simulink model "Application_Problem_Solution"  (R2018b)
settings: Solver=VariableStepAuto  StartTime=0.0  StopTime=6300  FixedStep=0.1  RelTol=1e-3  EnableMultiTasking=on
StopFcn:
  | if sum(Diagnostic_Decision_PV_1)>0
  | f = msgbox('Failure in PV 1');
  | end
  | 
  | if sum(Diagnostic_Decision_PV_2)>0
  | f = msgbox('Failure in PV 2');
  | end
  | 
  | if sum(Diagnostic_Decision_PV_3)>0
  | f = msgbox('Failure in PV 3');
  | end
  | 
  | if sum(Diagnostic_Decision_PV_4)>0
  | f = msgbox('Failure in PV 4');
  | end
  | 
  | if sum(Diagnostic_Decision_PV_5)>0
  | f = msgbox('Failure in PV 5');
  | end
  | 
  | if sum(Diagnostic_Decision_PV_6)>0
  | f = msgbox('Failure in PV 6');
  | end
  | 
  | if sum(Diagnostic_Decision_PV_7)>0
  | f = msgbox('Failure in PV 7');
  | end
  | 
  | if sum(Diagnostic_Decision_PV_8)>0
  | f = msgbox('Failure in PV 8');
  | end
  | 
  | if sum(Diagnostic_Decision_PV_9)>0
  | f = msgbox('Failure in PV 9');
  | end
  | 
  | if sum(Diagnostic_Decision_PV_10)>0
  | f = msgbox('Failure in PV 10');
  | end
values from neighbouring files (symbols this model uses):
  C1_LUT = [1913.6 4625.7 23306 10736 18036 12251 9022.9 12447 18872 40764 18721 33630 ... (21 elements, 7x3)]    [model_data_application.mat]
  Capacity_LUT = [28.0081 27.625 27.6392]    [model_data_application.mat]
  cell_Cp_heat = 810.5328    [model_data_application.mat]
  cell_mass = 1    [model_data_application.mat]
  Em_LUT = [3.4966 3.5519 3.6183 3.7066 3.9131 4.0748 4.1923 3.5057 3.566 3.6337 3.7127 3.9259 ... (21 elements, 7x3)]    [model_data_application.mat]
  Qe_init = 3.6845    [model_data_application.mat]
  R0_LUT = [0.0117 0.011 0.0114 0.0107 0.0107 0.0113 0.0116 0.0085 0.0085 0.0087 0.0082 0.0083 ... (21 elements, 7x3)]    [model_data_application.mat]
  R1_LUT = [0.0109 0.0069 0.0047 0.0034 0.0033 0.0033 0.0028 0.0029 0.0024 0.0026 0.0016 0.0023 ... (21 elements, 7x3)]    [model_data_application.mat]
  SOC_LUT = [0 0.1 0.25 0.5 0.75 0.9 1]    [model_data_application.mat]
  T_init = 293.15    [model_data_application.mat]
  Temperature_LUT = [278.15 293.15 313.15]    [model_data_application.mat]
undefined symbols (not defined in the file or in its folder): DiscIntNeverNeededParam
libraries: elec_lib x450, fl_lib x121, LiBatteryElements_lib x40, nesl_utility x32, simulink x10
(part 1 of 3)
settings Model: Creator=Sanjay Lodwal  LastModifiedBy=user
settings DataIOCC: LimitDataPoints=on  SaveFormat=Array
settings OptimizationCC: LifeSpan=inf
settings DebuggingCC: UnderspecifiedInitializationDetection=Classic  MergeDetectMultiDrivingBlocksExec=none  SolverPrmCheckMsg=warning  StateNameClashWarn=warning  SFUnexpectedBacktrackingDiag=warning  SFNoUnconditionalDefaultTransitionDiag=warning  SFExecutionAtInitializationDiag=none
settings HardwareCC: ProdBitPerPointer=32  ProdBitPerSizeT=32  ProdBitPerPtrDiffT=32  ProdLargestAtomicFloat=None  ProdIntDivRoundTo=Undefined  ProdEndianess=Unspecified  ProdWordSize=32  ProdHWDeviceType=32-bit Generic
settings ModelReferenceCC: PropagateSignalLabelsOutOfModel=off
settings SFSimCC: SimUseLocalCustomCode=off
settings RTWCC: RTWUseLocalCustomCode=off
settings CodeAppCC: StateflowObjectComments=on
settings GRTTargetCC: TargetLangStandard=C89/C90 (ANSI)  GeneratePreprocessorConditionals=Disable all
settings ConfigComp: CovMetricSettings=dw  CovHtmlReporting=on  CovSaveCumulativeToWorkspaceVar=on  CovSaveSingleToWorkspaceVar=on  CovExternalEMLEnable=off
settings SimscapeCC: SimscapeNormalizeSystem=off

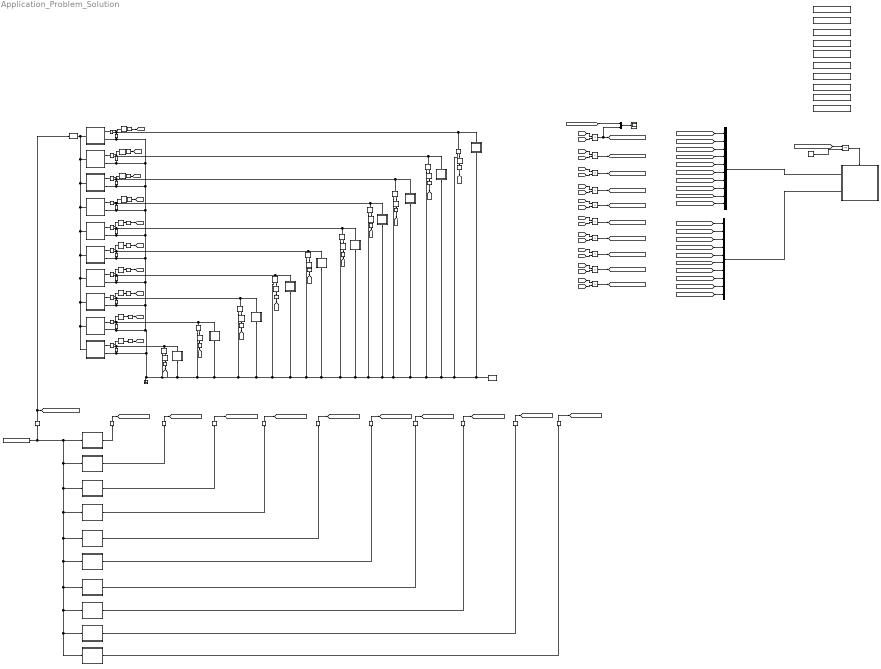
== system Application_Problem_Solution ==
  Battery1 : Subsystem  mask(Lithium cell (one RC-branch equivalent circuit)){Qe_init=Qe_init, T_init=T_init, Capacity_LUT=Capacity_LUT, Em_LUT=Em_LUT, R0_LUT=R0_LUT, R1_LUT=R1_LUT, C1_LUT=C1_LUT, cell_mass=cell_mass, cell_Cp_heat=cell_Cp_heat, SOC_LUT=SOC_LUT, Temperature_LUT=Temperature_LUT}
      mask prompts: Qe_init "Initial charge deficit (A*hr)"; T_init "Initial cell temperature (K)"; Capacity_LUT "Capacity (A*hr, 1xN table)"; Em_LUT "Em open-circuit voltage (volts, MxN table)"; R0_LUT "R0 terminal resistance (ohms, MxN table)"; R1_LUT "R1 resistance (ohms, MxN table)"; C1_LUT "C1 capacitance (farads, MxN table)"; cell_mass "Cell mass (kg)"; cell_Cp_heat "Cell specific heat (J/kg/K)"; SOC_LUT "SOC table breakpoints (Mx1 array)"; Temperature_LUT "Temperature table breakpoints (K, 1xN array)"
      mask DialogControl ParameterTabVar0 Prompt: Initial Conditions
      mask DialogControl ParameterTabVar01 Prompt: Electrical
      mask DialogControl ParameterTabVar012 Prompt: Thermal
      mask DialogControl ParameterTabVar0123 Prompt: Table Breakpoints
      mask Display: image('battery.jpg')
  Battery10 : Subsystem  mask(Lithium cell (one RC-branch equivalent circuit)){Qe_init=Qe_init, T_init=T_init, Capacity_LUT=Capacity_LUT, Em_LUT=Em_LUT, R0_LUT=R0_LUT, R1_LUT=R1_LUT, C1_LUT=C1_LUT, cell_mass=cell_mass, cell_Cp_heat=cell_Cp_heat, SOC_LUT=SOC_LUT, Temperature_LUT=Temperature_LUT}
      mask prompts: Qe_init "Initial charge deficit (A*hr)"; T_init "Initial cell temperature (K)"; Capacity_LUT "Capacity (A*hr, 1xN table)"; Em_LUT "Em open-circuit voltage (volts, MxN table)"; R0_LUT "R0 terminal resistance (ohms, MxN table)"; R1_LUT "R1 resistance (ohms, MxN table)"; C1_LUT "C1 capacitance (farads, MxN table)"; cell_mass "Cell mass (kg)"; cell_Cp_heat "Cell specific heat (J/kg/K)"; SOC_LUT "SOC table breakpoints (Mx1 array)"; Temperature_LUT "Temperature table breakpoints (K, 1xN array)"
      mask DialogControl ParameterTabVar0 Prompt: Initial Conditions
      mask DialogControl ParameterTabVar01 Prompt: Electrical
      mask DialogControl ParameterTabVar012 Prompt: Thermal
      mask DialogControl ParameterTabVar0123 Prompt: Table Breakpoints
      mask Display: image('battery.jpg')
  Battery2 : Subsystem  mask(Lithium cell (one RC-branch equivalent circuit)){Qe_init=Qe_init, T_init=T_init, Capacity_LUT=Capacity_LUT, Em_LUT=Em_LUT, R0_LUT=R0_LUT, R1_LUT=R1_LUT, C1_LUT=C1_LUT, cell_mass=cell_mass, cell_Cp_heat=cell_Cp_heat, SOC_LUT=SOC_LUT, Temperature_LUT=Temperature_LUT}
      mask prompts: Qe_init "Initial charge deficit (A*hr)"; T_init "Initial cell temperature (K)"; Capacity_LUT "Capacity (A*hr, 1xN table)"; Em_LUT "Em open-circuit voltage (volts, MxN table)"; R0_LUT "R0 terminal resistance (ohms, MxN table)"; R1_LUT "R1 resistance (ohms, MxN table)"; C1_LUT "C1 capacitance (farads, MxN table)"; cell_mass "Cell mass (kg)"; cell_Cp_heat "Cell specific heat (J/kg/K)"; SOC_LUT "SOC table breakpoints (Mx1 array)"; Temperature_LUT "Temperature table breakpoints (K, 1xN array)"
      mask DialogControl ParameterTabVar0 Prompt: Initial Conditions
      mask DialogControl ParameterTabVar01 Prompt: Electrical
      mask DialogControl ParameterTabVar012 Prompt: Thermal
      mask DialogControl ParameterTabVar0123 Prompt: Table Breakpoints
      mask Display: image('battery.jpg')
  Battery3 : Subsystem  mask(Lithium cell (one RC-branch equivalent circuit)){Qe_init=Qe_init, T_init=T_init, Capacity_LUT=Capacity_LUT, Em_LUT=Em_LUT, R0_LUT=R0_LUT, R1_LUT=R1_LUT, C1_LUT=C1_LUT, cell_mass=cell_mass, cell_Cp_heat=cell_Cp_heat, SOC_LUT=SOC_LUT, Temperature_LUT=Temperature_LUT}
      mask prompts: Qe_init "Initial charge deficit (A*hr)"; T_init "Initial cell temperature (K)"; Capacity_LUT "Capacity (A*hr, 1xN table)"; Em_LUT "Em open-circuit voltage (volts, MxN table)"; R0_LUT "R0 terminal resistance (ohms, MxN table)"; R1_LUT "R1 resistance (ohms, MxN table)"; C1_LUT "C1 capacitance (farads, MxN table)"; cell_mass "Cell mass (kg)"; cell_Cp_heat "Cell specific heat (J/kg/K)"; SOC_LUT "SOC table breakpoints (Mx1 array)"; Temperature_LUT "Temperature table breakpoints (K, 1xN array)"
      mask DialogControl ParameterTabVar0 Prompt: Initial Conditions
      mask DialogControl ParameterTabVar01 Prompt: Electrical
      mask DialogControl ParameterTabVar012 Prompt: Thermal
      mask DialogControl ParameterTabVar0123 Prompt: Table Breakpoints
      mask Display: image('battery.jpg')
  Battery4 : Subsystem  mask(Lithium cell (one RC-branch equivalent circuit)){Qe_init=Qe_init, T_init=T_init, Capacity_LUT=Capacity_LUT, Em_LUT=Em_LUT, R0_LUT=R0_LUT, R1_LUT=R1_LUT, C1_LUT=C1_LUT, cell_mass=cell_mass, cell_Cp_heat=cell_Cp_heat, SOC_LUT=SOC_LUT, Temperature_LUT=Temperature_LUT}
      mask prompts: Qe_init "Initial charge deficit (A*hr)"; T_init "Initial cell temperature (K)"; Capacity_LUT "Capacity (A*hr, 1xN table)"; Em_LUT "Em open-circuit voltage (volts, MxN table)"; R0_LUT "R0 terminal resistance (ohms, MxN table)"; R1_LUT "R1 resistance (ohms, MxN table)"; C1_LUT "C1 capacitance (farads, MxN table)"; cell_mass "Cell mass (kg)"; cell_Cp_heat "Cell specific heat (J/kg/K)"; SOC_LUT "SOC table breakpoints (Mx1 array)"; Temperature_LUT "Temperature table breakpoints (K, 1xN array)"
      mask DialogControl ParameterTabVar0 Prompt: Initial Conditions
      mask DialogControl ParameterTabVar01 Prompt: Electrical
      mask DialogControl ParameterTabVar012 Prompt: Thermal
      mask DialogControl ParameterTabVar0123 Prompt: Table Breakpoints
      mask Display: image('battery.jpg')
  Battery5 : Subsystem  mask(Lithium cell (one RC-branch equivalent circuit)){Qe_init=Qe_init, T_init=T_init, Capacity_LUT=Capacity_LUT, Em_LUT=Em_LUT, R0_LUT=R0_LUT, R1_LUT=R1_LUT, C1_LUT=C1_LUT, cell_mass=cell_mass, cell_Cp_heat=cell_Cp_heat, SOC_LUT=SOC_LUT, Temperature_LUT=Temperature_LUT}
      mask prompts: Qe_init "Initial charge deficit (A*hr)"; T_init "Initial cell temperature (K)"; Capacity_LUT "Capacity (A*hr, 1xN table)"; Em_LUT "Em open-circuit voltage (volts, MxN table)"; R0_LUT "R0 terminal resistance (ohms, MxN table)"; R1_LUT "R1 resistance (ohms, MxN table)"; C1_LUT "C1 capacitance (farads, MxN table)"; cell_mass "Cell mass (kg)"; cell_Cp_heat "Cell specific heat (J/kg/K)"; SOC_LUT "SOC table breakpoints (Mx1 array)"; Temperature_LUT "Temperature table breakpoints (K, 1xN array)"
      mask DialogControl ParameterTabVar0 Prompt: Initial Conditions
      mask DialogControl ParameterTabVar01 Prompt: Electrical
      mask DialogControl ParameterTabVar012 Prompt: Thermal
      mask DialogControl ParameterTabVar0123 Prompt: Table Breakpoints
      mask Display: image('battery.jpg')
  Battery6 : Subsystem  mask(Lithium cell (one RC-branch equivalent circuit)){Qe_init=Qe_init, T_init=T_init, Capacity_LUT=Capacity_LUT, Em_LUT=Em_LUT, R0_LUT=R0_LUT, R1_LUT=R1_LUT, C1_LUT=C1_LUT, cell_mass=cell_mass, cell_Cp_heat=cell_Cp_heat, SOC_LUT=SOC_LUT, Temperature_LUT=Temperature_LUT}
      mask prompts: Qe_init "Initial charge deficit (A*hr)"; T_init "Initial cell temperature (K)"; Capacity_LUT "Capacity (A*hr, 1xN table)"; Em_LUT "Em open-circuit voltage (volts, MxN table)"; R0_LUT "R0 terminal resistance (ohms, MxN table)"; R1_LUT "R1 resistance (ohms, MxN table)"; C1_LUT "C1 capacitance (farads, MxN table)"; cell_mass "Cell mass (kg)"; cell_Cp_heat "Cell specific heat (J/kg/K)"; SOC_LUT "SOC table breakpoints (Mx1 array)"; Temperature_LUT "Temperature table breakpoints (K, 1xN array)"
      mask DialogControl ParameterTabVar0 Prompt: Initial Conditions
      mask DialogControl ParameterTabVar01 Prompt: Electrical
      mask DialogControl ParameterTabVar012 Prompt: Thermal
      mask DialogControl ParameterTabVar0123 Prompt: Table Breakpoints
      mask Display: image('battery.jpg')
  Battery7 : Subsystem  mask(Lithium cell (one RC-branch equivalent circuit)){Qe_init=Qe_init, T_init=T_init, Capacity_LUT=Capacity_LUT, Em_LUT=Em_LUT, R0_LUT=R0_LUT, R1_LUT=R1_LUT, C1_LUT=C1_LUT, cell_mass=cell_mass, cell_Cp_heat=cell_Cp_heat, SOC_LUT=SOC_LUT, Temperature_LUT=Temperature_LUT}
      mask prompts: Qe_init "Initial charge deficit (A*hr)"; T_init "Initial cell temperature (K)"; Capacity_LUT "Capacity (A*hr, 1xN table)"; Em_LUT "Em open-circuit voltage (volts, MxN table)"; R0_LUT "R0 terminal resistance (ohms, MxN table)"; R1_LUT "R1 resistance (ohms, MxN table)"; C1_LUT "C1 capacitance (farads, MxN table)"; cell_mass "Cell mass (kg)"; cell_Cp_heat "Cell specific heat (J/kg/K)"; SOC_LUT "SOC table breakpoints (Mx1 array)"; Temperature_LUT "Temperature table breakpoints (K, 1xN array)"
      mask DialogControl ParameterTabVar0 Prompt: Initial Conditions
      mask DialogControl ParameterTabVar01 Prompt: Electrical
      mask DialogControl ParameterTabVar012 Prompt: Thermal
      mask DialogControl ParameterTabVar0123 Prompt: Table Breakpoints
      mask Display: image('battery.jpg')
  Battery8 : Subsystem  mask(Lithium cell (one RC-branch equivalent circuit)){Qe_init=Qe_init, T_init=T_init, Capacity_LUT=Capacity_LUT, Em_LUT=Em_LUT, R0_LUT=R0_LUT, R1_LUT=R1_LUT, C1_LUT=C1_LUT, cell_mass=cell_mass, cell_Cp_heat=cell_Cp_heat, SOC_LUT=SOC_LUT, Temperature_LUT=Temperature_LUT}
      mask prompts: Qe_init "Initial charge deficit (A*hr)"; T_init "Initial cell temperature (K)"; Capacity_LUT "Capacity (A*hr, 1xN table)"; Em_LUT "Em open-circuit voltage (volts, MxN table)"; R0_LUT "R0 terminal resistance (ohms, MxN table)"; R1_LUT "R1 resistance (ohms, MxN table)"; C1_LUT "C1 capacitance (farads, MxN table)"; cell_mass "Cell mass (kg)"; cell_Cp_heat "Cell specific heat (J/kg/K)"; SOC_LUT "SOC table breakpoints (Mx1 array)"; Temperature_LUT "Temperature table breakpoints (K, 1xN array)"
      mask DialogControl ParameterTabVar0 Prompt: Initial Conditions
      mask DialogControl ParameterTabVar01 Prompt: Electrical
      mask DialogControl ParameterTabVar012 Prompt: Thermal
      mask DialogControl ParameterTabVar0123 Prompt: Table Breakpoints
      mask Display: image('battery.jpg')
  Battery9 : Subsystem  mask(Lithium cell (one RC-branch equivalent circuit)){Qe_init=Qe_init, T_init=T_init, Capacity_LUT=Capacity_LUT, Em_LUT=Em_LUT, R0_LUT=R0_LUT, R1_LUT=R1_LUT, C1_LUT=C1_LUT, cell_mass=cell_mass, cell_Cp_heat=cell_Cp_heat, SOC_LUT=SOC_LUT, Temperature_LUT=Temperature_LUT}
      mask prompts: Qe_init "Initial charge deficit (A*hr)"; T_init "Initial cell temperature (K)"; Capacity_LUT "Capacity (A*hr, 1xN table)"; Em_LUT "Em open-circuit voltage (volts, MxN table)"; R0_LUT "R0 terminal resistance (ohms, MxN table)"; R1_LUT "R1 resistance (ohms, MxN table)"; C1_LUT "C1 capacitance (farads, MxN table)"; cell_mass "Cell mass (kg)"; cell_Cp_heat "Cell specific heat (J/kg/K)"; SOC_LUT "SOC table breakpoints (Mx1 array)"; Temperature_LUT "Temperature table breakpoints (K, 1xN array)"
      mask DialogControl ParameterTabVar0 Prompt: Initial Conditions
      mask DialogControl ParameterTabVar01 Prompt: Electrical
      mask DialogControl ParameterTabVar012 Prompt: Thermal
      mask DialogControl ParameterTabVar0123 Prompt: Table Breakpoints
      mask Display: image('battery.jpg')
  Current Sensor{,1..9} (10 alike) : fl_lib/Electrical/Electrical Sensors/Current Sensor
  Data Store Memory : DataStoreMemory  DataStoreName=Diagnostic_Decision_PV_1  ReadBeforeWriteMsg=warning  WriteAfterWriteMsg=warning  WriteAfterReadMsg=warning  ShowAdditionalParam=off
  Data Store Memory1 : DataStoreMemory  DataStoreName=Diagnostic_Decision_PV_2  ReadBeforeWriteMsg=warning  WriteAfterWriteMsg=warning  WriteAfterReadMsg=warning  ShowAdditionalParam=off
  Data Store Memory2 : DataStoreMemory  DataStoreName=Diagnostic_Decision_PV_3  ReadBeforeWriteMsg=warning  WriteAfterWriteMsg=warning  WriteAfterReadMsg=warning  ShowAdditionalParam=off
  Data Store Memory3 : DataStoreMemory  DataStoreName=Diagnostic_Decision_PV_4  ReadBeforeWriteMsg=warning  WriteAfterWriteMsg=warning  WriteAfterReadMsg=warning  ShowAdditionalParam=off
  Data Store Memory4 : DataStoreMemory  DataStoreName=Diagnostic_Decision_PV_5  ReadBeforeWriteMsg=warning  WriteAfterWriteMsg=warning  WriteAfterReadMsg=warning  ShowAdditionalParam=off
  Data Store Memory5 : DataStoreMemory  DataStoreName=Diagnostic_Decision_PV_6  ReadBeforeWriteMsg=warning  WriteAfterWriteMsg=warning  WriteAfterReadMsg=warning  ShowAdditionalParam=off
  Data Store Memory6 : DataStoreMemory  DataStoreName=Diagnostic_Decision_PV_7  ReadBeforeWriteMsg=warning  WriteAfterWriteMsg=warning  WriteAfterReadMsg=warning  ShowAdditionalParam=off
  Data Store Memory7 : DataStoreMemory  DataStoreName=Diagnostic_Decision_PV_8  ReadBeforeWriteMsg=warning  WriteAfterWriteMsg=warning  WriteAfterReadMsg=warning  ShowAdditionalParam=off
  Data Store Memory8 : DataStoreMemory  DataStoreName=Diagnostic_Decision_PV_9  ReadBeforeWriteMsg=warning  WriteAfterWriteMsg=warning  WriteAfterReadMsg=warning  ShowAdditionalParam=off
  Data Store Memory9 : DataStoreMemory  DataStoreName=Diagnostic_Decision_PV_10  ReadBeforeWriteMsg=warning  WriteAfterWriteMsg=warning  WriteAfterReadMsg=warning  ShowAdditionalParam=off
  Diagnostic Block : Subsystem  TreatAsAtomicUnit=on
  Diode{,1..9} (10 alike) : fl_lib/Electrical/Electrical Elements/Diode  Vf=0.6 V  Ron=0.3 Ohm  Goff=1e-8 1/Ohm  i_specify=off  i_priority=High  i=0 A  i_nominal_specify=off  i_nominal_unit=A  i_nominal_value=1  v_specify=off  v_priority=High  v=0 V  v_nominal_specify=off  v_nominal_unit=V  v_nominal_value=1
  Electrical Reference : fl_lib/Electrical/Electrical Elements/Electrical Reference
  Ir : FromWorkspace  VariableName=irradiance_measurement_8hrs  SampleTime=0
  Minimum Light Conditions : Constant  Value=500
  Mux : Mux  Inputs=2
  Mux1 : Mux  Inputs=10
  Mux2 : Mux  Inputs=10
  PS-Simulink Converter{1..20} (20 alike) : nesl_utility/PS-Simulink Converter  PhysicalDomain=network_engine_domain  SubClassName=ps_output  LeftPortType=input  RightPortType=output  PseudoPeriodic=off  Frequencies=[]  Unit=1  AffineConversion=off
  PV 1 Physical : Subsystem
      mask Display: image('PV_physical.png');
  PV 10 Physical : Subsystem
      mask Display: image('PV_physical.png');
  "PV 2 Physical " : Subsystem
      mask Display: image('PV_physical.png');
  PV 3 Physical : Subsystem
      mask Display: image('PV_physical.png');
  PV 4 Physical : Subsystem
      mask Display: image('PV_physical.png');
  PV 5 Physical : Subsystem
      mask Display: image('PV_physical.png');
  PV 6 Physical : Subsystem
      mask Display: image('PV_physical.png');
  PV 7 Physical : Subsystem
      mask Display: image('PV_physical.png');
  PV 8 Physical : Subsystem
      mask Display: image('PV_physical.png');
  PV 9 Physical : Subsystem
      mask Display: image('PV_physical.png');
  PV1 Digital Twin : Subsystem  mask{Isc=5.49, Voc=21.5, n=1.5, Rs=0, Ir0=1000, T=30}
      mask prompts: Isc "Short circuit current"; Voc "Open circuit voltage"; n "Quality factor, N"; Rs "Series resistance"; Ir0 "Reference irradiation"; T "Temperature"
      mask Display: image('PV1.jpg')
  PV10 Digital Twin : Subsystem  mask{Isc=5.49, Voc=21.5, n=1.5, Rs=0, Ir0=1000, T=30}
      mask prompts: Isc "Short circuit current"; Voc "Open circuit voltage"; n "Quality factor, N"; Rs "Series resistance"; Ir0 "Reference irradiation"; T "Temperature"
      mask Display: image('PV1.jpg')
  PV2 Digital Twin : Subsystem  mask{Isc=5.49, Voc=21.5, n=1.5, Rs=0, Ir0=1000, T=30}
      mask prompts: Isc "Short circuit current"; Voc "Open circuit voltage"; n "Quality factor, N"; Rs "Series resistance"; Ir0 "Reference irradiation"; T "Temperature"
      mask Display: image('PV1.jpg')
  "PV3 Digital Twin " : Subsystem  mask{Isc=5.49, Voc=21.5, n=1.5, Rs=0, Ir0=1000, T=30}
      mask prompts: Isc "Short circuit current"; Voc "Open circuit voltage"; n "Quality factor, N"; Rs "Series resistance"; Ir0 "Reference irradiation"; T "Temperature"
      mask Display: image('PV1.jpg')
  PV4 Digital Twin : Subsystem  mask{Isc=5.49, Voc=21.5, n=1.5, Rs=0, Ir0=1000, T=30}
      mask prompts: Isc "Short circuit current"; Voc "Open circuit voltage"; n "Quality factor, N"; Rs "Series resistance"; Ir0 "Reference irradiation"; T "Temperature"
      mask Display: image('PV1.jpg')
  PV5 Digital Twin : Subsystem  mask{Isc=5.49, Voc=21.5, n=1.5, Rs=0, Ir0=1000, T=30}
      mask prompts: Isc "Short circuit current"; Voc "Open circuit voltage"; n "Quality factor, N"; Rs "Series resistance"; Ir0 "Reference irradiation"; T "Temperature"
      mask Display: image('PV1.jpg')
  PV6 Digital Twin : Subsystem  mask{Isc=5.49, Voc=21.5, n=1.5, Rs=0, Ir0=1000, T=30}
      mask prompts: Isc "Short circuit current"; Voc "Open circuit voltage"; n "Quality factor, N"; Rs "Series resistance"; Ir0 "Reference irradiation"; T "Temperature"
      mask Display: image('PV1.jpg')
  PV7 Digital Twin : Subsystem  mask{Isc=5.49, Voc=21.5, n=1.5, Rs=0, Ir0=1000, T=30}
      mask prompts: Isc "Short circuit current"; Voc "Open circuit voltage"; n "Quality factor, N"; Rs "Series resistance"; Ir0 "Reference irradiation"; T "Temperature"
      mask Display: image('PV1.jpg')
  PV8 Digital Twin : Subsystem  mask{Isc=5.49, Voc=21.5, n=1.5, Rs=0, Ir0=1000, T=30}
      mask prompts: Isc "Short circuit current"; Voc "Open circuit voltage"; n "Quality factor, N"; Rs "Series resistance"; Ir0 "Reference irradiation"; T "Temperature"
      mask Display: image('PV1.jpg')
  PV9 Digital Twin : Subsystem  mask{Isc=5.49, Voc=21.5, n=1.5, Rs=0, Ir0=1000, T=30}
      mask prompts: Isc "Short circuit current"; Voc "Open circuit voltage"; n "Quality factor, N"; Rs "Series resistance"; Ir0 "Reference irradiation"; T "Temperature"
      mask Display: image('PV1.jpg')
  Product{,1..9} (10 alike) : Product
  Relational Operator : RelationalOperator  OutDataTypeStr=boolean  RndMeth=Simplest
  Scope : Scope
  Simulink-PS Converter1 : nesl_utility/Simulink-PS Converter  PhysicalDomain=network_engine_domain  SubClassName=ps_input  LeftPortType=input  RightPortType=output  PseudoPeriodic=off  Frequencies=[]  NoiseDistribution=none  NoiseParameters=[]  Unit=1  AffineConversion=off  FilteringAndDerivatives=zero  SimscapeFilterOrder=1  InputFilterTimeConstant=0.001  UdotUserProvided=1
  Solver Configuration : nesl_utility/Solver Configuration  PhysicalDomain=network_engine_domain  SubClassName=solver  LeftPortType=input  RightPortType=generic  Tones=[]  Harmonics=[]  SimulateNoise=off  Profile=off  UseLocalSampling=off  EnableSwitchedLinearOptims=on  FrequencyDomain=off  UseCCode=off  RelTol=0.001  AbsTol=1e-06  MinStep=1e-09  ToWorkspace=off  RevertToSquareIcSolve=off  NumHomotopyIterations=100  PhasorMode=off  PhasorModeNumHarmonics=1  DoDC=off  ResidualTolerance=1e-09  UseLocalSolver=off  LocalSolverChoice=NE_BACKWARD_EULER_ADVANCER  LocalSolverSampleTime=0.001  DoFixedCost=off  MaxNonlinIter=3  MaxModeIter=2  LinearAlgebra=Sparse  EquationFormulation=NE_TIME_EF  DelaysMemoryBudget=1024  AutomaticFiltering=on  FilteringTimeConstant=0.001  PartitionStorageMethod=AS_NEEDED  PartitionMemoryBudget=1024
  Voltage Sensor{1..3,7..13} (10 alike) : fl_lib/Electrical/Electrical Sensors/Voltage Sensor
  Zero-Order Hold{,1..30} (31 alike) : ZeroOrderHold  SampleTime=10
  wires:
  [I1] -> Product/1
  [V1] -> Product/2
  Product/1 -> [Power_PV1_digital_twin], Mux/2
  Product1/1 -> [Power_PV2_digital_twin]
  [V2] -> Product1/2
  [I2] -> Product1/1
  [I3] -> Product2/1
  [V3] -> Product2/2
  Product2/1 -> [Power_PV3_digital_twin]
  Product3/1 -> [Power_PV4_digital_twin]
  [V4] -> Product3/2
  [I4] -> Product3/1
  [I5] -> Product4/1
  [V5] -> Product4/2
  Product4/1 -> [Power_PV5_digital_twin]
  Product5/1 -> [Power_PV6_digital_twin]
  [V6] -> Product5/2
  [I6] -> Product5/1
  [I7] -> Product6/1
  [V7] -> Product6/2
  Product6/1 -> [Power_PV7_digital_twin]
  Product7/1 -> [Power_PV8_digital_twin]
  [V8] -> Product7/2
  [I8] -> Product7/1
  [I9] -> Product8/1
  [V9] -> Product8/2
  Product8/1 -> [Power_PV9_digital_twin]
  Product9/1 -> [Power_PV10_digital_twin]
  [V10] -> Product9/2
  [I10] -> Product9/1
  Zero-Order Hold/1 -> [I1]
  PS-Simulink Converter3/1 -> Zero-Order Hold/1
  PS-Simulink Converter1/1 -> Zero-Order Hold1/1
  Zero-Order Hold1/1 -> [I2]
  PS-Simulink Converter2/1 -> Zero-Order Hold2/1
  Zero-Order Hold2/1 -> [I3]
  Zero-Order Hold3/1 -> [I4]
  PS-Simulink Converter4/1 -> Zero-Order Hold3/1
  PS-Simulink Converter5/1 -> Zero-Order Hold4/1
  Zero-Order Hold4/1 -> [I5]
  Zero-Order Hold5/1 -> [I6]
  PS-Simulink Converter6/1 -> Zero-Order Hold5/1
  PS-Simulink Converter7/1 -> Zero-Order Hold6/1
  Zero-Order Hold6/1 -> [I7]
  PS-Simulink Converter8/1 -> Zero-Order Hold7/1
  Zero-Order Hold7/1 -> [I8]
  Zero-Order Hold8/1 -> [I9]
  PS-Simulink Converter9/1 -> Zero-Order Hold8/1
  Zero-Order Hold9/1 -> [I10]
  PS-Simulink Converter10/1 -> Zero-Order Hold9/1
  Zero-Order Hold10/1 -> [V10]
  PS-Simulink Converter20/1 -> Zero-Order Hold10/1
  PS-Simulink Converter19/1 -> Zero-Order Hold11/1
  Zero-Order Hold11/1 -> [V9]
  PS-Simulink Converter18/1 -> Zero-Order Hold12/1
  Zero-Order Hold12/1 -> [V8]
  PS-Simulink Converter17/1 -> Zero-Order Hold13/1
  Zero-Order Hold13/1 -> [V7]
  PS-Simulink Converter16/1 -> Zero-Order Hold14/1
  Zero-Order Hold14/1 -> [V6]
  PS-Simulink Converter15/1 -> Zero-Order Hold15/1
  Zero-Order Hold15/1 -> [V5]
  Zero-Order Hold16/1 -> [V4]
  PS-Simulink Converter14/1 -> Zero-Order Hold16/1
  PS-Simulink Converter13/1 -> Zero-Order Hold17/1
  Zero-Order Hold17/1 -> [V3]
  PS-Simulink Converter12/1 -> Zero-Order Hold18/1
  Zero-Order Hold18/1 -> [V2]
  PS-Simulink Converter11/1 -> Zero-Order Hold19/1
  Zero-Order Hold19/1 -> [V1]
  Ir/1 -> PV 10 Physical/1(In1), PV 9 Physical/1(In1), PV 8 Physical/1(In1), PV 7 Physical/1(In1), PV 6 Physical/1(In1), PV 5 Physical/1(In1), PV 4 Physical/1(In1), PV 3 Physical/1(In1), "PV 2 Physical "/1(In1), PV 1 Physical/1(In1), Zero-Order Hold20/1
  Zero-Order Hold20/1 -> Simulink-PS Converter1/1, [irradiance_measurement]
  PV 1 Physical/1(Out1) -> Zero-Order Hold21/1
  "PV 2 Physical "/1(Out1) -> Zero-Order Hold22/1
  PV 3 Physical/1(Out1) -> Zero-Order Hold23/1
  PV 4 Physical/1(Out1) -> Zero-Order Hold24/1
  PV 5 Physical/1(Out1) -> Zero-Order Hold25/1
  PV 6 Physical/1(Out1) -> Zero-Order Hold26/1
  PV 7 Physical/1(Out1) -> Zero-Order Hold27/1
  PV 8 Physical/1(Out1) -> Zero-Order Hold28/1
  PV 9 Physical/1(Out1) -> Zero-Order Hold29/1
  PV 10 Physical/1(Out1) -> Zero-Order Hold30/1
  [Power_PV1_physical_asset] -> Mux/1
  Mux/1 -> Scope/1
  [irradiance_measurement] -> Relational Operator/1
  Minimum Light Conditions/1 -> Relational Operator/2
  Relational Operator/1 -> Diagnostic Block/Enable
  Zero-Order Hold21/1 -> [Power_PV1_physical_asset]
  Zero-Order Hold22/1 -> [Power_PV2_physical_asset]
  Zero-Order Hold23/1 -> [Power_PV3_physical_asset]
  Zero-Order Hold24/1 -> [Power_PV4_physical_asset]
  Zero-Order Hold25/1 -> [Power_PV5_physical_asset]
  Zero-Order Hold26/1 -> [Power_PV6_physical_asset]
  Zero-Order Hold27/1 -> [Power_PV7_physical_asset]
  Zero-Order Hold28/1 -> [Power_PV8_physical_asset]
  Zero-Order Hold29/1 -> [Power_PV9_physical_asset]
  Zero-Order Hold30/1 -> [Power_PV10_physical_asset]
  [Power_PV8_physical_asset] -> Mux1/8
  [Power_PV9_physical_asset] -> Mux1/9
  [Power_PV6_physical_asset] -> Mux1/6
  [Power_PV7_physical_asset] -> Mux1/7
  [Power_PV10_physical_asset] -> Mux1/10
  [Power_PV4_physical_asset] -> Mux1/4
  [Power_PV5_physical_asset] -> Mux1/5
  [Power_PV2_physical_asset] -> Mux1/2
  [Power_PV3_physical_asset] -> Mux1/3
  [Power_PV1_physical_asset] -> Mux1/1
  [Power_PV2_digital_twin] -> Mux2/2
  [Power_PV7_digital_twin] -> Mux2/7
  [Power_PV8_digital_twin] -> Mux2/8
  [Power_PV1_digital_twin] -> Mux2/1
  [Power_PV3_digital_twin] -> Mux2/3
  [Power_PV5_digital_twin] -> Mux2/5
  [Power_PV6_digital_twin] -> Mux2/6
  [Power_PV9_digital_twin] -> Mux2/9
  [Power_PV10_digital_twin] -> Mux2/10
  [Power_PV4_digital_twin] -> Mux2/4
  Mux2/1 -> Diagnostic Block/2(Digital Twin PV-Power)
  Mux1/1 -> Diagnostic Block/1(Physical PV-Power)
  connections:
  Simulink-PS Converter1/RConn1 -- PV10 Digital Twin/LConn1 -- PV9 Digital Twin/LConn1 -- PV8 Digital Twin/LConn1 -- PV7 Digital Twin/LConn1 -- PV6 Digital Twin/LConn1 -- PV5 Digital Twin/LConn1 -- PV4 Digital Twin/LConn1 -- "PV3 Digital Twin "/LConn1 -- PV2 Digital Twin/LConn1 -- PV1 Digital Twin/LConn1
  Voltage Sensor1/LConn1 -- Diode/RConn1 -- Current Sensor/RConn2 -- Battery1/LConn1
  Diode1/RConn1 -- Battery2/LConn1 -- Voltage Sensor2/LConn1 -- Current Sensor1/RConn2
  Current Sensor/LConn1 -- PV1 Digital Twin/RConn1
  PV2 Digital Twin/RConn1 -- Current Sensor1/LConn1
  Diode2/RConn1 -- Current Sensor2/RConn2 -- Voltage Sensor3/LConn1 -- Battery3/LConn1
  Current Sensor3/RConn2 -- Diode3/RConn1 -- Battery4/LConn1 -- Voltage Sensor7/LConn1
  PV5 Digital Twin/RConn1 -- Current Sensor4/LConn1
  Diode4/RConn1 -- Current Sensor4/RConn2 -- Battery5/LConn1 -- Voltage Sensor8/LConn1
  Current Sensor5/RConn2 -- Diode5/RConn1 -- Battery6/LConn1 -- Voltage Sensor9/LConn1
  Diode6/RConn1 -- Current Sensor6/RConn2 -- Battery7/LConn1 -- Voltage Sensor10/LConn1
  Current Sensor7/RConn2 -- Diode7/RConn1 -- Voltage Sensor11/LConn1 -- Battery8/LConn1
  PV9 Digital Twin/RConn1 -- Current Sensor8/LConn1
  Diode8/RConn1 -- Current Sensor8/RConn2 -- Battery9/LConn1 -- Voltage Sensor12/LConn1
  Current Sensor9/RConn2 -- Diode9/RConn1 -- Battery10/LConn1 -- Voltage Sensor13/LConn1
  Current Sensor/RConn1 -- PS-Simulink Converter3/LConn1
  Current Sensor1/RConn1 -- PS-Simulink Converter1/LConn1
  Current Sensor2/RConn1 -- PS-Simulink Converter2/LConn1
  PS-Simulink Converter4/LConn1 -- Current Sensor3/RConn1
  PS-Simulink Converter5/LConn1 -- Current Sensor4/RConn1
  PS-Simulink Converter6/LConn1 -- Current Sensor5/RConn1
  PS-Simulink Converter7/LConn1 -- Current Sensor6/RConn1
  PS-Simulink Converter8/LConn1 -- Current Sensor7/RConn1
  PS-Simulink Converter9/LConn1 -- Current Sensor8/RConn1
  PS-Simulink Converter10/LConn1 -- Current Sensor9/RConn1
  Voltage Sensor1/RConn1 -- PS-Simulink Converter11/LConn1
  Voltage Sensor2/RConn1 -- PS-Simulink Converter12/LConn1
  Voltage Sensor3/RConn1 -- PS-Simulink Converter13/LConn1
  Voltage Sensor7/RConn1 -- PS-Simulink Converter14/LConn1
  Voltage Sensor8/RConn1 -- PS-Simulink Converter15/LConn1
  Voltage Sensor9/RConn1 -- PS-Simulink Converter16/LConn1
  Voltage Sensor10/RConn1 -- PS-Simulink Converter17/LConn1
  Voltage Sensor11/RConn1 -- PS-Simulink Converter18/LConn1
  Voltage Sensor12/RConn1 -- PS-Simulink Converter19/LConn1
  Diode/LConn1 -- PV1 Digital Twin/RConn2 -- Electrical Reference/LConn1 -- Battery10/RConn1 -- Voltage Sensor12/RConn2 -- Voltage Sensor8/RConn2 -- Voltage Sensor2/RConn2 -- Solver Configuration/RConn1 -- Battery1/RConn1 -- Voltage Sensor1/RConn2 -- Battery2/RConn1 -- Battery3/RConn1 -- Voltage Sensor3/RConn2 -- Battery4/RConn1 -- Voltage Sensor7/RConn2 -- Battery5/RConn1 -- Battery6/RConn1 -- Voltage Sensor9/RConn2 -- Battery7/RConn1 -- Voltage Sensor10/RConn2 -- Battery8/RConn1 -- Voltage Sensor11/RConn2 -- Battery9/RConn1 -- Voltage Sensor13/RConn2 -- PV10 Digital Twin/RConn2 -- Diode9/LConn1 -- Diode8/LConn1 -- PV9 Digital Twin/RConn2 -- Diode7/LConn1 -- PV8 Digital Twin/RConn2 -- Diode6/LConn1 -- PV7 Digital Twin/RConn2 -- PV6 Digital Twin/RConn2 -- Diode5/LConn1 -- PV5 Digital Twin/RConn2 -- Diode4/LConn1 -- PV4 Digital Twin/RConn2 -- Diode3/LConn1 -- Diode2/LConn1 -- "PV3 Digital Twin "/RConn2 -- PV2 Digital Twin/RConn2 -- Diode1/LConn1
  Voltage Sensor13/RConn1 -- PS-Simulink Converter20/LConn1
  "PV3 Digital Twin "/RConn1 -- Current Sensor2/LConn1
  PV4 Digital Twin/RConn1 -- Current Sensor3/LConn1
  PV6 Digital Twin/RConn1 -- Current Sensor5/LConn1
  PV7 Digital Twin/RConn1 -- Current Sensor6/LConn1
  PV10 Digital Twin/RConn1 -- Current Sensor9/LConn1
  PV8 Digital Twin/RConn1 -- Current Sensor7/LConn1

== system Application_Problem_Solution/Battery1 ==
  C1 : LiBatteryElements_lib/C_table  C_Table=C1_LUT F  SOC_Table=SOC_LUT  Temp_Table=Temperature_LUT K  v0=0 V
  Convective Heat Transfer : fl_lib/Thermal/Thermal Elements/Convective Heat Transfer  area=cell_area m^2  heat_tr_coeff=h_conv W/(m^2 * K)  T_specify=off  T_priority=High  T=0 K  T_nominal_specify=off  T_nominal_unit=K  T_nominal_value=1  Q_specify=off  Q_priority=High  Q=0 J/s  Q_nominal_specify=off  Q_nominal_unit=W  Q_nominal_value=1
  Em_table : LiBatteryElements_lib/Em_table  C_Table=Capacity_LUT hr*A  Em_Table=Em_LUT V  SOC_Table=SOC_LUT  Temp_Table=Temperature_LUT K  Qinit=Qe_init hr*A
  Ideal Temperature Source : fl_lib/Thermal/Thermal Sources/Controlled Temperature Source
      settings: SourceProductName=Simscape
  Power Sum : fl_lib/Physical Signals/Functions/PS Add
  R0 : LiBatteryElements_lib/R_table  R_Table=R0_LUT Ohm  SOC_Table=SOC_LUT  Temp_Table=Temperature_LUT K
  R1 : LiBatteryElements_lib/R_table  R_Table=R1_LUT Ohm  SOC_Table=SOC_LUT  Temp_Table=Temperature_LUT K
  Simulink-PS Converter2 : nesl_utility/Simulink-PS Converter  PhysicalDomain=network_engine_domain  SubClassName=ps_input  LeftPortType=input  RightPortType=output  PseudoPeriodic=off  Frequencies=[]  NoiseDistribution=none  NoiseParameters=[]  Unit=degC  AffineConversion=on  FilteringAndDerivatives=zero  SimscapeFilterOrder=1  InputFilterTimeConstant=.001  UdotUserProvided=1
  Thermal Model : Subsystem
  Thermal Reference : fl_lib/Thermal/Thermal Elements/Thermal Reference
  temp : Constant  Value=25
  + : PMIOPort  Tag=PMCPort  Side=Left
  - : PMIOPort  Tag=PMCPort  Port=2  Side=Right
  wires:
  temp/1 -> Simulink-PS Converter2/1
  connections:
  R1/LConn3 -- R0/LConn3 -- Em_table/LConn3 -- C1/LConn3
  Convective Heat Transfer/RConn1 -- Thermal Model/LConn2
  Em_table/RConn1 -- -/RConn1
  +/RConn1 -- R0/RConn1
  Em_table/LConn1 -- C1/LConn1 -- R1/LConn1
  R1/RConn2 -- Power Sum/LConn2
  R1/LConn2 -- Thermal Model/RConn1 -- Em_table/RConn2 -- R0/LConn2 -- C1/LConn2
  Power Sum/RConn1 -- Thermal Model/LConn1
  R1/RConn1 -- C1/RConn1 -- R0/LConn1
  R0/RConn2 -- Power Sum/LConn1
  Simulink-PS Converter2/RConn1 -- Ideal Temperature Source/RConn1
  Ideal Temperature Source/LConn1 -- Convective Heat Transfer/LConn1
  Thermal Reference/LConn1 -- Ideal Temperature Source/RConn2

== system Application_Problem_Solution/Battery10 ==
  C1 : LiBatteryElements_lib/C_table  C_Table=C1_LUT F  SOC_Table=SOC_LUT  Temp_Table=Temperature_LUT K  v0=0 V
  Convective Heat Transfer : fl_lib/Thermal/Thermal Elements/Convective Heat Transfer  area=cell_area m^2  heat_tr_coeff=h_conv W/(m^2 * K)  T_specify=off  T_priority=High  T=0 K  T_nominal_specify=off  T_nominal_unit=K  T_nominal_value=1  Q_specify=off  Q_priority=High  Q=0 J/s  Q_nominal_specify=off  Q_nominal_unit=W  Q_nominal_value=1
  Em_table : LiBatteryElements_lib/Em_table  C_Table=Capacity_LUT hr*A  Em_Table=Em_LUT V  SOC_Table=SOC_LUT  Temp_Table=Temperature_LUT K  Qinit=Qe_init hr*A
  Ideal Temperature Source : fl_lib/Thermal/Thermal Sources/Controlled Temperature Source
      settings: SourceProductName=Simscape
  Power Sum : fl_lib/Physical Signals/Functions/PS Add
  R0 : LiBatteryElements_lib/R_table  R_Table=R0_LUT Ohm  SOC_Table=SOC_LUT  Temp_Table=Temperature_LUT K
  R1 : LiBatteryElements_lib/R_table  R_Table=R1_LUT Ohm  SOC_Table=SOC_LUT  Temp_Table=Temperature_LUT K
  Simulink-PS Converter2 : nesl_utility/Simulink-PS Converter  PhysicalDomain=network_engine_domain  SubClassName=ps_input  LeftPortType=input  RightPortType=output  PseudoPeriodic=off  Frequencies=[]  NoiseDistribution=none  NoiseParameters=[]  Unit=degC  AffineConversion=on  FilteringAndDerivatives=zero  SimscapeFilterOrder=1  InputFilterTimeConstant=.001  UdotUserProvided=1
  Thermal Model : Subsystem
  Thermal Reference : fl_lib/Thermal/Thermal Elements/Thermal Reference
  temp : Constant  Value=25
  + : PMIOPort  Tag=PMCPort  Side=Left
  - : PMIOPort  Tag=PMCPort  Port=2  Side=Right
  wires:
  temp/1 -> Simulink-PS Converter2/1
  connections:
  R1/LConn3 -- R0/LConn3 -- Em_table/LConn3 -- C1/LConn3
  Convective Heat Transfer/RConn1 -- Thermal Model/LConn2
  Em_table/RConn1 -- -/RConn1
  +/RConn1 -- R0/RConn1
  Em_table/LConn1 -- C1/LConn1 -- R1/LConn1
  R1/RConn2 -- Power Sum/LConn2
  R1/LConn2 -- Thermal Model/RConn1 -- Em_table/RConn2 -- R0/LConn2 -- C1/LConn2
  Power Sum/RConn1 -- Thermal Model/LConn1
  R1/RConn1 -- C1/RConn1 -- R0/LConn1
  R0/RConn2 -- Power Sum/LConn1
  Simulink-PS Converter2/RConn1 -- Ideal Temperature Source/RConn1
  Ideal Temperature Source/LConn1 -- Convective Heat Transfer/LConn1
  Thermal Reference/LConn1 -- Ideal Temperature Source/RConn2

== system Application_Problem_Solution/Battery2 ==
  C1 : LiBatteryElements_lib/C_table  C_Table=C1_LUT F  SOC_Table=SOC_LUT  Temp_Table=Temperature_LUT K  v0=0 V
  Convective Heat Transfer : fl_lib/Thermal/Thermal Elements/Convective Heat Transfer  area=cell_area m^2  heat_tr_coeff=h_conv W/(m^2 * K)  T_specify=off  T_priority=High  T=0 K  T_nominal_specify=off  T_nominal_unit=K  T_nominal_value=1  Q_specify=off  Q_priority=High  Q=0 J/s  Q_nominal_specify=off  Q_nominal_unit=W  Q_nominal_value=1
  Em_table : LiBatteryElements_lib/Em_table  C_Table=Capacity_LUT hr*A  Em_Table=Em_LUT V  SOC_Table=SOC_LUT  Temp_Table=Temperature_LUT K  Qinit=Qe_init hr*A
  Ideal Temperature Source : fl_lib/Thermal/Thermal Sources/Controlled Temperature Source
      settings: SourceProductName=Simscape
  Power Sum : fl_lib/Physical Signals/Functions/PS Add
  R0 : LiBatteryElements_lib/R_table  R_Table=R0_LUT Ohm  SOC_Table=SOC_LUT  Temp_Table=Temperature_LUT K
  R1 : LiBatteryElements_lib/R_table  R_Table=R1_LUT Ohm  SOC_Table=SOC_LUT  Temp_Table=Temperature_LUT K
  Simulink-PS Converter2 : nesl_utility/Simulink-PS Converter  PhysicalDomain=network_engine_domain  SubClassName=ps_input  LeftPortType=input  RightPortType=output  PseudoPeriodic=off  Frequencies=[]  NoiseDistribution=none  NoiseParameters=[]  Unit=degC  AffineConversion=on  FilteringAndDerivatives=zero  SimscapeFilterOrder=1  InputFilterTimeConstant=.001  UdotUserProvided=1
  Thermal Model : Subsystem
  Thermal Reference : fl_lib/Thermal/Thermal Elements/Thermal Reference
  temp : Constant  Value=25
  + : PMIOPort  Tag=PMCPort  Side=Left
  - : PMIOPort  Tag=PMCPort  Port=2  Side=Right
  wires:
  temp/1 -> Simulink-PS Converter2/1
  connections:
  R1/LConn3 -- R0/LConn3 -- Em_table/LConn3 -- C1/LConn3
  Convective Heat Transfer/RConn1 -- Thermal Model/LConn2
  Em_table/RConn1 -- -/RConn1
  +/RConn1 -- R0/RConn1
  Em_table/LConn1 -- C1/LConn1 -- R1/LConn1
  R1/RConn2 -- Power Sum/LConn2
  R1/LConn2 -- Thermal Model/RConn1 -- Em_table/RConn2 -- R0/LConn2 -- C1/LConn2
  Power Sum/RConn1 -- Thermal Model/LConn1
  R1/RConn1 -- C1/RConn1 -- R0/LConn1
  R0/RConn2 -- Power Sum/LConn1
  Simulink-PS Converter2/RConn1 -- Ideal Temperature Source/RConn1
  Ideal Temperature Source/LConn1 -- Convective Heat Transfer/LConn1
  Thermal Reference/LConn1 -- Ideal Temperature Source/RConn2

== system Application_Problem_Solution/Battery3 ==
  C1 : LiBatteryElements_lib/C_table  C_Table=C1_LUT F  SOC_Table=SOC_LUT  Temp_Table=Temperature_LUT K  v0=0 V
  Convective Heat Transfer : fl_lib/Thermal/Thermal Elements/Convective Heat Transfer  area=cell_area m^2  heat_tr_coeff=h_conv W/(m^2 * K)  T_specify=off  T_priority=High  T=0 K  T_nominal_specify=off  T_nominal_unit=K  T_nominal_value=1  Q_specify=off  Q_priority=High  Q=0 J/s  Q_nominal_specify=off  Q_nominal_unit=W  Q_nominal_value=1
  Em_table : LiBatteryElements_lib/Em_table  C_Table=Capacity_LUT hr*A  Em_Table=Em_LUT V  SOC_Table=SOC_LUT  Temp_Table=Temperature_LUT K  Qinit=Qe_init hr*A
  Ideal Temperature Source : fl_lib/Thermal/Thermal Sources/Controlled Temperature Source
      settings: SourceProductName=Simscape
  Power Sum : fl_lib/Physical Signals/Functions/PS Add
  R0 : LiBatteryElements_lib/R_table  R_Table=R0_LUT Ohm  SOC_Table=SOC_LUT  Temp_Table=Temperature_LUT K
  R1 : LiBatteryElements_lib/R_table  R_Table=R1_LUT Ohm  SOC_Table=SOC_LUT  Temp_Table=Temperature_LUT K
  Simulink-PS Converter2 : nesl_utility/Simulink-PS Converter  PhysicalDomain=network_engine_domain  SubClassName=ps_input  LeftPortType=input  RightPortType=output  PseudoPeriodic=off  Frequencies=[]  NoiseDistribution=none  NoiseParameters=[]  Unit=degC  AffineConversion=on  FilteringAndDerivatives=zero  SimscapeFilterOrder=1  InputFilterTimeConstant=.001  UdotUserProvided=1
  Thermal Model : Subsystem
  Thermal Reference : fl_lib/Thermal/Thermal Elements/Thermal Reference
  temp : Constant  Value=25
  + : PMIOPort  Tag=PMCPort  Side=Left
  - : PMIOPort  Tag=PMCPort  Port=2  Side=Right
  wires:
  temp/1 -> Simulink-PS Converter2/1
  connections:
  Thermal Reference/LConn1 -- Ideal Temperature Source/RConn2
  Ideal Temperature Source/LConn1 -- Convective Heat Transfer/LConn1
  Simulink-PS Converter2/RConn1 -- Ideal Temperature Source/RConn1
  R0/RConn2 -- Power Sum/LConn1
  R0/LConn1 -- C1/RConn1 -- R1/RConn1
  Power Sum/RConn1 -- Thermal Model/LConn1
  C1/LConn2 -- R0/LConn2 -- Em_table/RConn2 -- Thermal Model/RConn1 -- R1/LConn2
  R1/RConn2 -- Power Sum/LConn2
  R1/LConn1 -- C1/LConn1 -- Em_table/LConn1
  +/RConn1 -- R0/RConn1
  Em_table/RConn1 -- -/RConn1
  Convective Heat Transfer/RConn1 -- Thermal Model/LConn2
  C1/LConn3 -- Em_table/LConn3 -- R0/LConn3 -- R1/LConn3

== system Application_Problem_Solution/Battery4 ==
  C1 : LiBatteryElements_lib/C_table  C_Table=C1_LUT F  SOC_Table=SOC_LUT  Temp_Table=Temperature_LUT K  v0=0 V
  Convective Heat Transfer : fl_lib/Thermal/Thermal Elements/Convective Heat Transfer  area=cell_area m^2  heat_tr_coeff=h_conv W/(m^2 * K)  T_specify=off  T_priority=High  T=0 K  T_nominal_specify=off  T_nominal_unit=K  T_nominal_value=1  Q_specify=off  Q_priority=High  Q=0 J/s  Q_nominal_specify=off  Q_nominal_unit=W  Q_nominal_value=1
  Em_table : LiBatteryElements_lib/Em_table  C_Table=Capacity_LUT hr*A  Em_Table=Em_LUT V  SOC_Table=SOC_LUT  Temp_Table=Temperature_LUT K  Qinit=Qe_init hr*A
  Ideal Temperature Source : fl_lib/Thermal/Thermal Sources/Controlled Temperature Source
      settings: SourceProductName=Simscape
  Power Sum : fl_lib/Physical Signals/Functions/PS Add
  R0 : LiBatteryElements_lib/R_table  R_Table=R0_LUT Ohm  SOC_Table=SOC_LUT  Temp_Table=Temperature_LUT K
  R1 : LiBatteryElements_lib/R_table  R_Table=R1_LUT Ohm  SOC_Table=SOC_LUT  Temp_Table=Temperature_LUT K
  Simulink-PS Converter2 : nesl_utility/Simulink-PS Converter  PhysicalDomain=network_engine_domain  SubClassName=ps_input  LeftPortType=input  RightPortType=output  PseudoPeriodic=off  Frequencies=[]  NoiseDistribution=none  NoiseParameters=[]  Unit=degC  AffineConversion=on  FilteringAndDerivatives=zero  SimscapeFilterOrder=1  InputFilterTimeConstant=.001  UdotUserProvided=1
  Thermal Model : Subsystem
  Thermal Reference : fl_lib/Thermal/Thermal Elements/Thermal Reference
  temp : Constant  Value=25
  + : PMIOPort  Tag=PMCPort  Side=Left
  - : PMIOPort  Tag=PMCPort  Port=2  Side=Right
  wires:
  temp/1 -> Simulink-PS Converter2/1
  connections:
  R1/LConn3 -- R0/LConn3 -- Em_table/LConn3 -- C1/LConn3
  Convective Heat Transfer/RConn1 -- Thermal Model/LConn2
  Em_table/RConn1 -- -/RConn1
  +/RConn1 -- R0/RConn1
  Em_table/LConn1 -- C1/LConn1 -- R1/LConn1
  R1/RConn2 -- Power Sum/LConn2
  R1/LConn2 -- Thermal Model/RConn1 -- Em_table/RConn2 -- R0/LConn2 -- C1/LConn2
  Power Sum/RConn1 -- Thermal Model/LConn1
  R1/RConn1 -- C1/RConn1 -- R0/LConn1
  R0/RConn2 -- Power Sum/LConn1
  Simulink-PS Converter2/RConn1 -- Ideal Temperature Source/RConn1
  Ideal Temperature Source/LConn1 -- Convective Heat Transfer/LConn1
  Thermal Reference/LConn1 -- Ideal Temperature Source/RConn2

== system Application_Problem_Solution/Battery5 ==
  C1 : LiBatteryElements_lib/C_table  C_Table=C1_LUT F  SOC_Table=SOC_LUT  Temp_Table=Temperature_LUT K  v0=0 V
  Convective Heat Transfer : fl_lib/Thermal/Thermal Elements/Convective Heat Transfer  area=cell_area m^2  heat_tr_coeff=h_conv W/(m^2 * K)  T_specify=off  T_priority=High  T=0 K  T_nominal_specify=off  T_nominal_unit=K  T_nominal_value=1  Q_specify=off  Q_priority=High  Q=0 J/s  Q_nominal_specify=off  Q_nominal_unit=W  Q_nominal_value=1
  Em_table : LiBatteryElements_lib/Em_table  C_Table=Capacity_LUT hr*A  Em_Table=Em_LUT V  SOC_Table=SOC_LUT  Temp_Table=Temperature_LUT K  Qinit=Qe_init hr*A
  Ideal Temperature Source : fl_lib/Thermal/Thermal Sources/Controlled Temperature Source
      settings: SourceProductName=Simscape
  Power Sum : fl_lib/Physical Signals/Functions/PS Add
  R0 : LiBatteryElements_lib/R_table  R_Table=R0_LUT Ohm  SOC_Table=SOC_LUT  Temp_Table=Temperature_LUT K
  R1 : LiBatteryElements_lib/R_table  R_Table=R1_LUT Ohm  SOC_Table=SOC_LUT  Temp_Table=Temperature_LUT K
  Simulink-PS Converter2 : nesl_utility/Simulink-PS Converter  PhysicalDomain=network_engine_domain  SubClassName=ps_input  LeftPortType=input  RightPortType=output  PseudoPeriodic=off  Frequencies=[]  NoiseDistribution=none  NoiseParameters=[]  Unit=degC  AffineConversion=on  FilteringAndDerivatives=zero  SimscapeFilterOrder=1  InputFilterTimeConstant=.001  UdotUserProvided=1
  Thermal Model : Subsystem
  Thermal Reference : fl_lib/Thermal/Thermal Elements/Thermal Reference
  temp : Constant  Value=25
  + : PMIOPort  Tag=PMCPort  Side=Left
  - : PMIOPort  Tag=PMCPort  Port=2  Side=Right
  wires:
  temp/1 -> Simulink-PS Converter2/1
  connections:
  Thermal Reference/LConn1 -- Ideal Temperature Source/RConn2
  Ideal Temperature Source/LConn1 -- Convective Heat Transfer/LConn1
  Simulink-PS Converter2/RConn1 -- Ideal Temperature Source/RConn1
  R0/RConn2 -- Power Sum/LConn1
  R0/LConn1 -- C1/RConn1 -- R1/RConn1
  Power Sum/RConn1 -- Thermal Model/LConn1
  C1/LConn2 -- R0/LConn2 -- Em_table/RConn2 -- Thermal Model/RConn1 -- R1/LConn2
  R1/RConn2 -- Power Sum/LConn2
  R1/LConn1 -- C1/LConn1 -- Em_table/LConn1
  +/RConn1 -- R0/RConn1
  Em_table/RConn1 -- -/RConn1
  Convective Heat Transfer/RConn1 -- Thermal Model/LConn2
  C1/LConn3 -- Em_table/LConn3 -- R0/LConn3 -- R1/LConn3

== system Application_Problem_Solution/Battery6 ==
  C1 : LiBatteryElements_lib/C_table  C_Table=C1_LUT F  SOC_Table=SOC_LUT  Temp_Table=Temperature_LUT K  v0=0 V
  Convective Heat Transfer : fl_lib/Thermal/Thermal Elements/Convective Heat Transfer  area=cell_area m^2  heat_tr_coeff=h_conv W/(m^2 * K)  T_specify=off  T_priority=High  T=0 K  T_nominal_specify=off  T_nominal_unit=K  T_nominal_value=1  Q_specify=off  Q_priority=High  Q=0 J/s  Q_nominal_specify=off  Q_nominal_unit=W  Q_nominal_value=1
  Em_table : LiBatteryElements_lib/Em_table  C_Table=Capacity_LUT hr*A  Em_Table=Em_LUT V  SOC_Table=SOC_LUT  Temp_Table=Temperature_LUT K  Qinit=Qe_init hr*A
  Ideal Temperature Source : fl_lib/Thermal/Thermal Sources/Controlled Temperature Source
      settings: SourceProductName=Simscape
  Power Sum : fl_lib/Physical Signals/Functions/PS Add
  R0 : LiBatteryElements_lib/R_table  R_Table=R0_LUT Ohm  SOC_Table=SOC_LUT  Temp_Table=Temperature_LUT K
  R1 : LiBatteryElements_lib/R_table  R_Table=R1_LUT Ohm  SOC_Table=SOC_LUT  Temp_Table=Temperature_LUT K
  Simulink-PS Converter2 : nesl_utility/Simulink-PS Converter  PhysicalDomain=network_engine_domain  SubClassName=ps_input  LeftPortType=input  RightPortType=output  PseudoPeriodic=off  Frequencies=[]  NoiseDistribution=none  NoiseParameters=[]  Unit=degC  AffineConversion=on  FilteringAndDerivatives=zero  SimscapeFilterOrder=1  InputFilterTimeConstant=.001  UdotUserProvided=1
  Thermal Model : Subsystem
  Thermal Reference : fl_lib/Thermal/Thermal Elements/Thermal Reference
  temp : Constant  Value=25
  + : PMIOPort  Tag=PMCPort  Side=Left
  - : PMIOPort  Tag=PMCPort  Port=2  Side=Right
  wires:
  temp/1 -> Simulink-PS Converter2/1
  connections:
  R1/LConn3 -- R0/LConn3 -- Em_table/LConn3 -- C1/LConn3
  Convective Heat Transfer/RConn1 -- Thermal Model/LConn2
  Em_table/RConn1 -- -/RConn1
  +/RConn1 -- R0/RConn1
  Em_table/LConn1 -- C1/LConn1 -- R1/LConn1
  R1/RConn2 -- Power Sum/LConn2
  R1/LConn2 -- Thermal Model/RConn1 -- Em_table/RConn2 -- R0/LConn2 -- C1/LConn2
  Power Sum/RConn1 -- Thermal Model/LConn1
  R1/RConn1 -- C1/RConn1 -- R0/LConn1
  R0/RConn2 -- Power Sum/LConn1
  Simulink-PS Converter2/RConn1 -- Ideal Temperature Source/RConn1
  Ideal Temperature Source/LConn1 -- Convective Heat Transfer/LConn1
  Thermal Reference/LConn1 -- Ideal Temperature Source/RConn2
